simulink model "EC_prioridad"  (R2023b)
settings: Solver=VariableStepAuto  StartTime=0.0  StopTime=25  RelTol=1e-3
undefined symbols (not defined in the file or in its folder): m, n
settings Model: Creator=anruk  LastModifiedBy=anruk

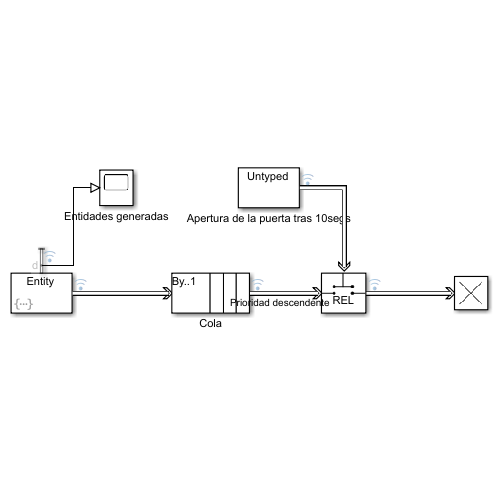
[thumbnail: Simulink's stored preview of the top-level diagram]
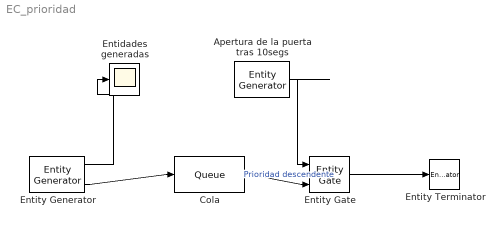
== system EC_prioridad ==
  Apertura de la puerta tras 10segs : EntityGenerator  OutputPortMessageModes=m  TimeSource=MATLAB action  IntergenerationTimeAction=|  GenerateEntityAtSimulationStart=off  AttributeName=entity  AttributeInitialValue=0  EntityTypeName=Entity
      | % Cada valor de la secuencia representa el retardo en liberar las entidades
      | % de la cola
      | persistent SEC;
      | persistent idx;
      | if isempty(SEC)
      | SEC = [10 1 1 1 1 1 1 1 1 1];
      | idx = 1;
      | end
      | if idx > numel(SEC)
      | dt= inf;
      | else
      | dt = SEC(idx);
      | end
      | idx = idx + 1;
  Cola : Queue  InputPortMessageModes=m  OutputPortMessageModes=m  QueueType=Priority  PrioritySource=Atributo1  SortingDirection=Descending
  Entidades generadas : Scope
  Entity Gate : EntityGate  InputPortMessageModes=m,m  OutputPortMessageModes=m  OperatingMode=Release gate
  Entity Generator : EntityGenerator  OutputPortMessageModes=n,m  TimeSource=MATLAB action  IntergenerationTimeAction=|  GenerateEntityAtSimulationStart=off  GenerateAction=|  AttributeName=Atributo1  NumberEntitiesDeparted=on  EntityType=Structured  EntityTypeName=Entity
      IntergenerationTimeAction=|
      | % Patrón de repetición de secuencia
      | % Se inicializan las variables
      | persistent SEC;
      | persistent idx;
      | if isempty(SEC)
      | % Se generan 10 entidades con 1 segundo de intervalo
      | SEC = [1 1 1 1 1 1 1 1 1 1];
      | idx = 1;
      | end
      | if idx > numel(SEC)
      | % Se detiene la generación de entidades después de 10
      | dt = inf;
      | else
      | dt = SEC(idx);
      | end
      | idx = idx + 1;
      GenerateAction=|
      | % Se modifica el valor del atributo de la entidad en cada paso de reloj.
      | persistent SEC1;
      | persistent idx1;
      | if isempty(SEC1)
      | SEC1 = [1 2 3 4 5 6 7 8 9 10];
      | idx1 = 1;
      | end
      | if idx1 <= numel(SEC1)
      | entity.Atributo1 = SEC1(idx1);
      | end
      | idx1 = idx1 + 1;
      settings: OutputPortMap=o0,o3
  Entity Terminator : EntityTerminator  InputPortMessageModes=m
  wires:
  Entity Gate/1 -> Entity Terminator/1
  Cola/1 -> Entity Gate/2  "Prioridad descendente"
  Entity Generator/1 -> Entidades generadas/1
  Apertura de la puerta tras 10segs/1 -> Entity Gate/1
  Entity Generator/2 -> Cola/1
